simulink model "ROBOT4"  (R2019a)
settings: Solver=VariableStepAuto  StartTime=0.0  StopTime=inf  RelTol=1e-3
StartFcn:
  | 1
values from neighbouring files (symbols this model uses):
  s = sqrt((z4-a1)^2+r4^2)    [CONTROL.m]
undefined symbols (not defined in the file or in its folder): Base, Link1, Link2, Link3, Link4, ROBOT4, RootPart
libraries: mblibv1 x18, simulink x4
settings Model: Creator=MyPC  LastModifiedBy=csank
settings DataIOCC: ReturnWorkspaceOutputs=off
settings OptimizationCC: BlockReduction=off
settings DebuggingCC: ArithmeticOperatorsInVariantConditions=warning
settings SFSimCC: SimUseLocalCustomCode=off
settings RTWCC: RTWUseLocalCustomCode=off
settings CodeAppCC: StateflowObjectComments=on
settings SimscapeCC: SimscapeNormalizeSystem=off
settings SimMechanicsCC: VisOnUpdateDiagram=on  VisDuringSimulation=on

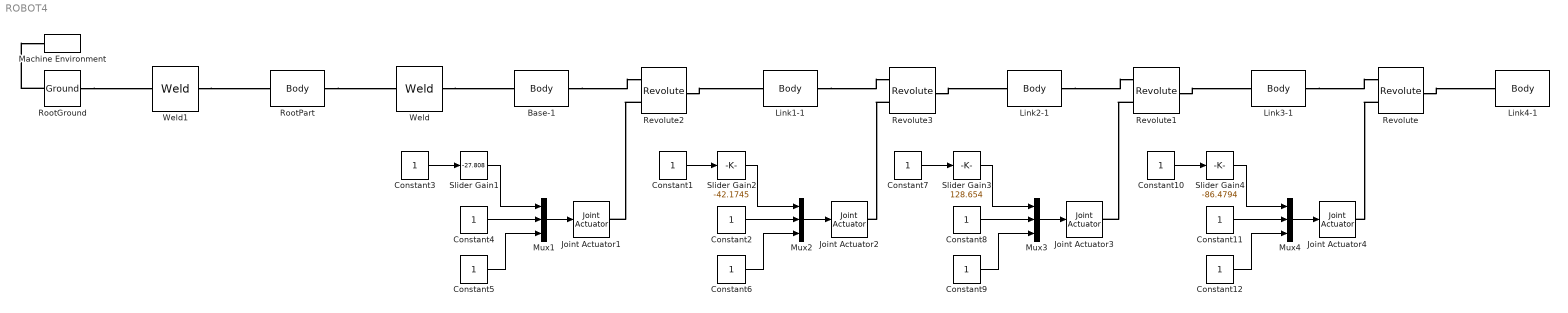
== system ROBOT4 ==
  Base-1 : mblibv1/Bodies/Body  LConnTagsString=CS2  RConnTagsString=CS3  UpdateFromCAD=on  PMImportedID=Base-1  DialogClass=MechanicalBodyBlock  Mass=20.055  MassUnits=kg  InertiaUnits=kg*m^2  Inertia=[0.425156,1.30045e-05,-3.32729e-05;1.30045e-05,0.499103,-0.0411844;-3.32729e-05,-0.0411844,0.340025]  Shape=Cylinder  ShapeDims=[1 1]  ShapeUnits=m  ShapeUse=false  Density=1  DensityUnits=kg/m^3  DensityUse=false  GraphicsMode=GFXFILE  GraphicsFileName=ROBOT4 - Base-1.STL  BodyColorSelMode=COLORPALETTE  BodyColor=[0.25098;0.25098;0.25098]  AttachedToCS=CS1  CG=Right$CG$[0.143839 0.24611 0.488748]$WORLD$WORLD$m$[1 0 0;0 1 0;0 0 1]$3x3 Transform$rad$WORLD$false$Base-1::CG(AUTOGEN)  WorkingFrames=Right$CS1$[0.143832 0.162841 0.457249]$WORLD$WORLD$m$[1 0 0;0 1 0;0 0 1]$3x3 Transform$rad$WORLD$false$Base-1::CS1(AUTOGEN)#Left$CS2$[0.143839 0.24611 0.488748]$WORLD$WORLD$m$[1 0 0;0 1 0;0 0 1]$3x3 Transform$rad$WORLD$true$Base-1:-:ROBOT4/RootPart::Base-1(AUTOGEN)#Right$CS3$[0.143832 0.312841 0.457249]$WORLD$WORLD$m$[1 0 0;0 1 0;0 0 1]$3x3 Transform$rad$WORLD$true$Base-1:-:Link1-1::Base-1(AUTOGEN)  CGPos=[0.143839 0.24611 0.488748]  CGRot=[1 0 0;0 1 0;0 0 1]  CS0Pos=[]  CS0Rot=[]  CS1Pos=[0.143832 0.162841 0.457249]  CS1Rot=[1 0 0;0 1 0;0 0 1]  CS2Pos=[0.143839 0.24611 0.488748]  CS2Rot=[1 0 0;0 1 0;0 0 1]  CS3Pos=[0.143832 0.312841 0.457249]  CS3Rot=[1 0 0;0 1 0;0 0 1]  CS4Pos=[]  CS4Rot=[]  CS5Pos=[]  CS5Rot=[]  CS6Pos=[]  CS6Rot=[]  CS7Pos=[]  CS7Rot=[]  CS8Pos=[]  CS8Rot=[]  CS9Pos=[]  CS9Rot=[]  CS10Pos=[]  CS10Rot=[]  CS11Pos=[]  CS11Rot=[]  CS12Pos=[]  CS12Rot=[]  CS13Pos=[]  CS13Rot=[]  CS14Pos=[]  CS14Rot=[]  CS15Pos=[]  CS15Rot=[]  CS16Pos=[]  CS16Rot=[]  CS17Pos=[]  CS17Rot=[]  CS18Pos=[]  CS18Rot=[]  CS19Pos=[]  CS19Rot=[]  CS20Pos=[]  CS20Rot=[]
      settings: SourceProductName=Simscape Multibody  SourceProductBaseCode=MS
  Constant{1..12} (12 alike) : Constant
  Joint Actuator{1..4} (4 alike) : mblibv1/Sensors &  Actuators/Joint Actuator  UpdateFromCAD=off  PhysicalDomain=Mechanical  PortType=blob  ActuationStyle=Motion  AngleUnits=deg  ArcVelocityUnits=deg/s  ArcAccelerationUnits=deg/s^2  CoordPositionUnits=m  VelocityUnits=m/s  AccelerationUnits=m/s^2  ForceUnits=N  TorqueUnits=N*m  ActiveIO=on  Width=3  DialogClass=MechanicalActuatorBlock  Primitive=R1  ReferenceFrame=Absolute (World)
      settings: SourceProductName=Simscape Multibody  SourceProductBaseCode=MS
  Link1-1 : mblibv1/Bodies/Body  LConnTagsString=CS2  RConnTagsString=CS3  UpdateFromCAD=on  PMImportedID=Link1-1  DialogClass=MechanicalBodyBlock  Mass=14.5082  MassUnits=kg  InertiaUnits=kg*m^2  Inertia=[0.281196,-1.21205e-09,1.25074e-09;-1.21205e-09,0.109377,0;1.25074e-09,0,0.307869]  Shape=Cylinder  ShapeDims=[1 1]  ShapeUnits=m  ShapeUse=false  Density=1  DensityUnits=kg/m^3  DensityUse=false  GraphicsMode=GFXFILE  GraphicsFileName=ROBOT4 - Link1-1.STL  BodyColorSelMode=COLORPALETTE  BodyColor=[0;0;1]  AttachedToCS=CS1  CG=Right$CG$[0.143832 0.525874 0.457249]$WORLD$WORLD$m$[0.791183 0 0.61158;0 1 0;-0.61158 0 0.791183]$3x3 Transform$rad$WORLD$false$Link1-1::CG(AUTOGEN)  WorkingFrames=Right$CS1$[0.143832 0.312841 0.457249]$WORLD$WORLD$m$[0.791183 0 0.61158;0 1 0;-0.61158 0 0.791183]$3x3 Transform$rad$WORLD$false$Link1-1::CS1(AUTOGEN)#Left$CS2$[0.143832 0.312841 0.457249]$WORLD$WORLD$m$[1 0 0;0 1 0;0 0 1]$3x3 Transform$rad$WORLD$true$Base-1:-:Link1-1::Link1-1(AUTOGEN)#Right$CS3$[0.0887895 0.648841 0.386043]$WORLD$WORLD$m$[1 0 0;0 1 0;0 0 1]$3x3 Transform$rad$WORLD$true$Link1-1:-:Link2-1::Link1-1(AUTOGEN)  CGPos=[0.143832 0.525874 0.457249]  CGRot=[0.791183 0 0.61158;0 1 0;-0.61158 0 0.791183]  CS0Pos=[]  CS0Rot=[]  CS1Pos=[0.143832 0.312841 0.457249]  CS1Rot=[0.791183 0 0.61158;0 1 0;-0.61158 0 0.791183]  CS2Pos=[0.143832 0.312841 0.457249]  CS2Rot=[1 0 0;0 1 0;0 0 1]  CS3Pos=[0.0887895 0.648841 0.386043]  CS3Rot=[1 0 0;0 1 0;0 0 1]  CS4Pos=[]  CS4Rot=[]  CS5Pos=[]  CS5Rot=[]  CS6Pos=[]  CS6Rot=[]  CS7Pos=[]  CS7Rot=[]  CS8Pos=[]  CS8Rot=[]  CS9Pos=[]  CS9Rot=[]  CS10Pos=[]  CS10Rot=[]  CS11Pos=[]  CS11Rot=[]  CS12Pos=[]  CS12Rot=[]  CS13Pos=[]  CS13Rot=[]  CS14Pos=[]  CS14Rot=[]  CS15Pos=[]  CS15Rot=[]  CS16Pos=[]  CS16Rot=[]  CS17Pos=[]  CS17Rot=[]  CS18Pos=[]  CS18Rot=[]  CS19Pos=[]  CS19Rot=[]  CS20Pos=[]  CS20Rot=[]
      settings: SourceProductName=Simscape Multibody  SourceProductBaseCode=MS
  Link2-1 : mblibv1/Bodies/Body  LConnTagsString=CS3  RConnTagsString=CS2  UpdateFromCAD=on  PMImportedID=Link2-1  DialogClass=MechanicalBodyBlock  Mass=15.1518  MassUnits=kg  InertiaUnits=kg*m^2  Inertia=[0.614194,-0.00012408,2.07767e-05;-0.00012408,0.151653,3.7792e-06;2.07767e-05,3.7792e-06,0.703306]  Shape=Cylinder  ShapeDims=[1 1]  ShapeUnits=m  ShapeUse=false  Density=1  DensityUnits=kg/m^3  DensityUse=false  GraphicsMode=GFXFILE  GraphicsFileName=ROBOT4 - Link2-1.STL  BodyColorSelMode=COLORPALETTE  BodyColor=[0;0;1]  AttachedToCS=CS1  CG=Right$CG$[0.293105 0.676583 0.341751]$WORLD$WORLD$m$[-0.61158 0.782776 0.11503;0 0.14539 -0.989374;-0.791183 -0.605082 -0.0889177]$3x3 Transform$rad$WORLD$false$Link2-1::CG(AUTOGEN)  WorkingFrames=Right$CS1$[0.143832 0.648841 0.457249]$WORLD$WORLD$m$[-0.61158 0.782776 0.11503;0 0.14539 -0.989374;-0.791183 -0.605082 -0.0889177]$3x3 Transform$rad$WORLD$false$Link2-1::CS1(AUTOGEN)#Right$CS2$[0.480177 0.721536 0.0835021]$WORLD$WORLD$m$[1 0 0;0 1 0;0 0 1]$3x3 Transform$rad$WORLD$true$Link2-1:-:Link3-1::Link2-1(AUTOGEN)#Left$CS3$[0.0887895 0.648841 0.386043]$WORLD$WORLD$m$[1 0 0;0 1 0;0 0 1]$3x3 Transform$rad$WORLD$true$Link1-1:-:Link2-1::Link2-1(AUTOGEN)  CGPos=[0.293105 0.676583 0.341751]  CGRot=[-0.61158 0.782776 0.11503;0 0.14539 -0.989374;-0.791183 -0.605082 -0.0889177]  CS0Pos=[]  CS0Rot=[]  CS1Pos=[0.143832 0.648841 0.457249]  CS1Rot=[-0.61158 0.782776 0.11503;0 0.14539 -0.989374;-0.791183 -0.605082 -0.0889177]  CS2Pos=[0.480177 0.721536 0.0835021]  CS2Rot=[1 0 0;0 1 0;0 0 1]  CS3Pos=[0.0887895 0.648841 0.386043]  CS3Rot=[1 0 0;0 1 0;0 0 1]  CS4Pos=[]  CS4Rot=[]  CS5Pos=[]  CS5Rot=[]  CS6Pos=[]  CS6Rot=[]  CS7Pos=[]  CS7Rot=[]  CS8Pos=[]  CS8Rot=[]  CS9Pos=[]  CS9Rot=[]  CS10Pos=[]  CS10Rot=[]  CS11Pos=[]  CS11Rot=[]  CS12Pos=[]  CS12Rot=[]  CS13Pos=[]  CS13Rot=[]  CS14Pos=[]  CS14Rot=[]  CS15Pos=[]  CS15Rot=[]  CS16Pos=[]  CS16Rot=[]  CS17Pos=[]  CS17Rot=[]  CS18Pos=[]  CS18Rot=[]  CS19Pos=[]  CS19Rot=[]  CS20Pos=[]  CS20Rot=[]
      settings: SourceProductName=Simscape Multibody  SourceProductBaseCode=MS
  Link3-1 : mblibv1/Bodies/Body  LConnTagsString=CS3  RConnTagsString=CS2  UpdateFromCAD=on  PMImportedID=Link3-1  DialogClass=MechanicalBodyBlock  Mass=11.44  MassUnits=kg  InertiaUnits=kg*m^2  Inertia=[0.316807,0,0;0,0.0703346,0.0335673;0,0.0335673,0.293359]  Shape=Cylinder  ShapeDims=[1 1]  ShapeUnits=m  ShapeUse=false  Density=1  DensityUnits=kg/m^3  DensityUse=false  GraphicsMode=GFXFILE  GraphicsFileName=ROBOT4 - Link3-1.STL  BodyColorSelMode=COLORPALETTE  BodyColor=[0;0;1]  AttachedToCS=CS1  CG=Right$CG$[0.65417 0.825127 0.0627608]$WORLD$WORLD$m$[-0.61158 0.783362 -0.110968;0 -0.140256 -0.990115;-0.791183 -0.605535 0.0857777]$3x3 Transform$rad$WORLD$false$Link3-1::CG(AUTOGEN)  WorkingFrames=Right$CS1$[0.53522 0.721536 0.154709]$WORLD$WORLD$m$[-0.61158 0.783362 -0.110968;0 -0.140256 -0.990115;-0.791183 -0.605535 0.0857777]$3x3 Transform$rad$WORLD$false$Link3-1::CS1(AUTOGEN)#Right$CS2$[0.891317 0.809701 -0.0573564]$WORLD$WORLD$m$[1 0 0;0 1 0;0 0 1]$3x3 Transform$rad$WORLD$true$Link3-1:-:Link4-1::Link3-1(AUTOGEN)#Left$CS3$[0.480177 0.721536 0.0835021]$WORLD$WORLD$m$[1 0 0;0 1 0;0 0 1]$3x3 Transform$rad$WORLD$true$Link2-1:-:Link3-1::Link3-1(AUTOGEN)  CGPos=[0.65417 0.825127 0.0627608]  CGRot=[-0.61158 0.783362 -0.110968;0 -0.140256 -0.990115;-0.791183 -0.605535 0.0857777]  CS0Pos=[]  CS0Rot=[]  CS1Pos=[0.53522 0.721536 0.154709]  CS1Rot=[-0.61158 0.783362 -0.110968;0 -0.140256 -0.990115;-0.791183 -0.605535 0.0857777]  CS2Pos=[0.891317 0.809701 -0.0573564]  CS2Rot=[1 0 0;0 1 0;0 0 1]  CS3Pos=[0.480177 0.721536 0.0835021]  CS3Rot=[1 0 0;0 1 0;0 0 1]  CS4Pos=[]  CS4Rot=[]  CS5Pos=[]  CS5Rot=[]  CS6Pos=[]  CS6Rot=[]  CS7Pos=[]  CS7Rot=[]  CS8Pos=[]  CS8Rot=[]  CS9Pos=[]  CS9Rot=[]  CS10Pos=[]  CS10Rot=[]  CS11Pos=[]  CS11Rot=[]  CS12Pos=[]  CS12Rot=[]  CS13Pos=[]  CS13Rot=[]  CS14Pos=[]  CS14Rot=[]  CS15Pos=[]  CS15Rot=[]  CS16Pos=[]  CS16Rot=[]  CS17Pos=[]  CS17Rot=[]  CS18Pos=[]  CS18Rot=[]  CS19Pos=[]  CS19Rot=[]  CS20Pos=[]  CS20Rot=[]
      settings: SourceProductName=Simscape Multibody  SourceProductBaseCode=MS
  Link4-1 : mblibv1/Bodies/Body  LConnTagsString=CS2  UpdateFromCAD=on  PMImportedID=Link4-1  DialogClass=MechanicalBodyBlock  Mass=1.35899  MassUnits=kg  InertiaUnits=kg*m^2  Inertia=[0.00780395,1.96668e-09,2.46591e-09;1.96668e-09,0.00251605,2.02055e-09;2.46591e-09,2.02055e-09,0.00833468]  Shape=Cylinder  ShapeDims=[1 1]  ShapeUnits=m  ShapeUse=false  Density=1  DensityUnits=kg/m^3  DensityUse=false  GraphicsMode=GFXFILE  GraphicsFileName=ROBOT4 - Link4-1.STL  BodyColorSelMode=COLORPALETTE  BodyColor=[1;1;1]  AttachedToCS=CS1  CG=Right$CG$[0.857915 0.812027 -0.0947335]$WORLD$WORLD$m$[-0.432065 -0.662789 -0.61158;-0.83772 0.5461 0;0.333984 0.512333 -0.791183]$3x3 Transform$rad$WORLD$false$Link4-1::CG(AUTOGEN)  WorkingFrames=Right$CS1$[0.940273 0.744169 -0.158395]$WORLD$WORLD$m$[-0.432065 -0.662789 -0.61158;-0.83772 0.5461 0;0.333984 0.512333 -0.791183]$3x3 Transform$rad$WORLD$false$Link4-1::CS1(AUTOGEN)#Left$CS2$[0.891317 0.809701 -0.0573564]$WORLD$WORLD$m$[1 0 0;0 1 0;0 0 1]$3x3 Transform$rad$WORLD$true$Link3-1:-:Link4-1::Link4-1(AUTOGEN)  CGPos=[0.857915 0.812027 -0.0947335]  CGRot=[-0.432065 -0.662789 -0.61158;-0.83772 0.5461 0;0.333984 0.512333 -0.791183]  CS0Pos=[]  CS0Rot=[]  CS1Pos=[0.940273 0.744169 -0.158395]  CS1Rot=[-0.432065 -0.662789 -0.61158;-0.83772 0.5461 0;0.333984 0.512333 -0.791183]  CS2Pos=[0.891317 0.809701 -0.0573564]  CS2Rot=[1 0 0;0 1 0;0 0 1]  CS3Pos=[]  CS3Rot=[]  CS4Pos=[]  CS4Rot=[]  CS5Pos=[]  CS5Rot=[]  CS6Pos=[]  CS6Rot=[]  CS7Pos=[]  CS7Rot=[]  CS8Pos=[]  CS8Rot=[]  CS9Pos=[]  CS9Rot=[]  CS10Pos=[]  CS10Rot=[]  CS11Pos=[]  CS11Rot=[]  CS12Pos=[]  CS12Rot=[]  CS13Pos=[]  CS13Rot=[]  CS14Pos=[]  CS14Rot=[]  CS15Pos=[]  CS15Rot=[]  CS16Pos=[]  CS16Rot=[]  CS17Pos=[]  CS17Rot=[]  CS18Pos=[]  CS18Rot=[]  CS19Pos=[]  CS19Rot=[]  CS20Pos=[]  CS20Rot=[]
      settings: SourceProductName=Simscape Multibody  SourceProductBaseCode=MS
  Machine Environment : mblibv1/Bodies/Machine Environment  PortType=env  PhysicalDomain=Mechanical  DialogTemplateClass=MECH.MachineEnvironment  SyncWhenCopied=off  Gravity=[0 -9.81 0]  GravityUnits=m/s^2  GravityAsSignal=off  Dimensionality=Auto-detect  AnalysisType=Forward dynamics  LinearAssemblyTolerance=1e-3  LinearAssemblyToleranceUnits=m  AngularAssemblyTolerance=1e-3  AngularAssemblyToleranceUnits=rad  ConstraintSolverType=Stabilizing  ConstraintRelTolerance=1e-4  ConstraintAbsTolerance=1e-4  UseRobustSingularityHandling=off  RedundancyAnalysisToleranceType=Automatically select tolerance  RedundancyAnalysisTolerance=1e-14  StatePerturbationType=Fixed  PerturbationSize=1e-5  VisualizeMachine=on  BodyVisualizationType=Use model default body geometries  BodyColorSelMode=Use model default  DefaultBodyColor=[1 0 0]
      settings: SourceProductName=Simscape Multibody  SourceProductBaseCode=MS
  Mux{1..4} (4 alike) : Mux  Inputs=3
  Revolute : mblibv1/Joints/Revolute  LConnTagsString=__newl0|SA1  RConnTagsString=__newr0  UpdateFromCAD=on  PMImportedID=Link3-1:-:Link4-1  NumSAPorts=1  CutJoint=off  MarkAsCut=off  Primitives=prismatic  PrimitiveProps=R1$World$[-0.61158,0,-0.791183]$revolute  DialogClass=JointBlock  R1Axis=[-0.61158,0,-0.791183]
      settings: SourceProductName=Simscape Multibody  SourceProductBaseCode=MS
  Revolute1 : mblibv1/Joints/Revolute  LConnTagsString=__newl0|SA1  RConnTagsString=__newr0  UpdateFromCAD=on  PMImportedID=Link2-1:-:Link3-1  NumSAPorts=1  CutJoint=off  MarkAsCut=off  Primitives=prismatic  PrimitiveProps=R1$World$[0.61158,0,0.791183]$revolute  DialogClass=JointBlock  R1Axis=[0.61158,0,0.791183]
      settings: SourceProductName=Simscape Multibody  SourceProductBaseCode=MS
  Revolute2 : mblibv1/Joints/Revolute  LConnTagsString=__newl0|SA1  RConnTagsString=__newr0  UpdateFromCAD=on  PMImportedID=Base-1:-:Link1-1  NumSAPorts=1  CutJoint=off  MarkAsCut=off  Primitives=prismatic  PrimitiveProps=R1$World$[0,1,0]$revolute  DialogClass=JointBlock  R1Axis=[0,1,0]
      settings: SourceProductName=Simscape Multibody  SourceProductBaseCode=MS
  Revolute3 : mblibv1/Joints/Revolute  LConnTagsString=__newl0|SA1  RConnTagsString=__newr0  UpdateFromCAD=on  PMImportedID=Link1-1:-:Link2-1  NumSAPorts=1  CutJoint=off  MarkAsCut=off  Primitives=prismatic  PrimitiveProps=R1$World$[-0.61158,0,-0.791183]$revolute  DialogClass=JointBlock  R1Axis=[-0.61158,0,-0.791183]
      settings: SourceProductName=Simscape Multibody  SourceProductBaseCode=MS
  RootGround : mblibv1/Bodies/Ground  UpdateFromCAD=on  PMImportedID=RootGround  LeftPortType=env  RightPortType=workingframe  PhysicalDomain=Mechanical  DialogClass=GroundBlock  CoordPosition=[0.288929,0.533635,0.35517]  CoordPositionUnits=m  StateVectorMgrId=0  MachineId=[1 0]  ShowEnvPort=on  ParameterChecksum=[2237965960, 2493805458, 3117988158, 3002818646]  TopologyChecksum=[2414812317, 896225707, 3049100628, 567793257]
      settings: SourceProductName=Simscape Multibody  SourceProductBaseCode=MS
  RootPart : mblibv1/Bodies/Body  LConnTagsString=CS3  RConnTagsString=CS2  UpdateFromCAD=on  PMImportedID=ROBOT4/RootPart  DialogClass=MechanicalBodyBlock  Mass=0  MassUnits=kg  InertiaUnits=kg*m^2  Inertia=[0,0,0;0,0,0;0,0,0]  Shape=Cylinder  ShapeDims=[1 1]  ShapeUnits=m  ShapeUse=false  Density=1  DensityUnits=kg/m^3  DensityUse=false  GraphicsMode=MACHINE_DEFAULT  BodyColorSelMode=MACHINE_DEFAULT  BodyColor=[1;0;0]  AttachedToCS=CS1  CG=Right$CG$[0.288929 0.533635 0.35517]$WORLD$WORLD$m$[1 0 0;0 1 0;0 0 1]$3x3 Transform$rad$WORLD$false$ROBOT4/RootPart::CG(AUTOGEN)  WorkingFrames=Right$CS1$[0 0 0]$WORLD$WORLD$m$[1 0 0;0 1 0;0 0 1]$3x3 Transform$rad$WORLD$false$ROBOT4/RootPart::CS1(AUTOGEN)#Right$CS2$[0.143839 0.24611 0.488748]$WORLD$WORLD$m$[1 0 0;0 1 0;0 0 1]$3x3 Transform$rad$WORLD$true$Base-1:-:ROBOT4/RootPart::ROBOT4/RootPart(AUTOGEN)#Left$CS3$[0.288929 0.533635 0.35517]$WORLD$WORLD$m$[1 0 0;0 1 0;0 0 1]$3x3 Transform$rad$WORLD$true$ROBOT4/RootPart:-:RootGround::ROBOT4/RootPart(AUTOGEN)  CGPos=[0.288929 0.533635 0.35517]  CGRot=[1 0 0;0 1 0;0 0 1]  CS0Pos=[]  CS0Rot=[]  CS1Pos=[0 0 0]  CS1Rot=[1 0 0;0 1 0;0 0 1]  CS2Pos=[0.143839 0.24611 0.488748]  CS2Rot=[1 0 0;0 1 0;0 0 1]  CS3Pos=[0.288929 0.533635 0.35517]  CS3Rot=[1 0 0;0 1 0;0 0 1]  CS4Pos=[]  CS4Rot=[]  CS5Pos=[]  CS5Rot=[]  CS6Pos=[]  CS6Rot=[]  CS7Pos=[]  CS7Rot=[]  CS8Pos=[]  CS8Rot=[]  CS9Pos=[]  CS9Rot=[]  CS10Pos=[]  CS10Rot=[]  CS11Pos=[]  CS11Rot=[]  CS12Pos=[]  CS12Rot=[]  CS13Pos=[]  CS13Rot=[]  CS14Pos=[]  CS14Rot=[]  CS15Pos=[]  CS15Rot=[]  CS16Pos=[]  CS16Rot=[]  CS17Pos=[]  CS17Rot=[]  CS18Pos=[]  CS18Rot=[]  CS19Pos=[]  CS19Rot=[]  CS20Pos=[]  CS20Rot=[]
      settings: SourceProductName=Simscape Multibody  SourceProductBaseCode=MS
  Slider Gain1 : simulink/Math Operations/Slider Gain  gain=-27.808  low=-180  high=180
  Slider Gain2 : simulink/Math Operations/Slider Gain  gain=-42.1745  low=-180  high=180
  Slider Gain3 : simulink/Math Operations/Slider Gain  gain=128.654  low=-180  high=180
  Slider Gain4 : simulink/Math Operations/Slider Gain  gain=-86.4794  low=-180  high=180
  Weld : mblibv1/Joints/Weld  LConnTagsString=__newl0  RConnTagsString=__newr0  UpdateFromCAD=on  PMImportedID=Base-1:-:ROBOT4/RootPart  NumSAPorts=0  CutJoint=off  MarkAsCut=off  Primitives=weld  PrimitiveProps=W$WORLD$[0.57735,0.57735,0.57735]$weld  DialogClass=JointBlock  WAxis=[0.57735,0.57735,0.57735]
      settings: SourceProductName=Simscape Multibody  SourceProductBaseCode=MS
  Weld1 : mblibv1/Joints/Weld  LConnTagsString=__newl0  RConnTagsString=__newr0  UpdateFromCAD=on  PMImportedID=ROBOT4/RootPart:-:RootGround  NumSAPorts=0  CutJoint=off  MarkAsCut=off  Primitives=weld  PrimitiveProps=W$WORLD$[0.57735,0.57735,0.57735]$weld  DialogClass=JointBlock  WAxis=[0.57735,0.57735,0.57735]
      settings: SourceProductName=Simscape Multibody  SourceProductBaseCode=MS
  wires:
  Slider Gain1/1 -> Mux1/1
  Mux1/1 -> Joint Actuator1/1
  Constant3/1 -> Slider Gain1/1
  Constant5/1 -> Mux1/3
  Constant4/1 -> Mux1/2
  Slider Gain2/1 -> Mux2/1
  Mux2/1 -> Joint Actuator2/1
  Constant1/1 -> Slider Gain2/1
  Constant6/1 -> Mux2/3
  Constant2/1 -> Mux2/2
  Slider Gain3/1 -> Mux3/1
  Mux3/1 -> Joint Actuator3/1
  Constant7/1 -> Slider Gain3/1
  Constant9/1 -> Mux3/3
  Constant8/1 -> Mux3/2
  Slider Gain4/1 -> Mux4/1
  Mux4/1 -> Joint Actuator4/1
  Constant10/1 -> Slider Gain4/1
  Constant12/1 -> Mux4/3
  Constant11/1 -> Mux4/2
  connections:
  RootPart/RConn1 -- Weld/LConn1
  Weld/RConn1 -- Base-1/LConn1
  Link3-1/RConn1 -- Revolute/LConn1
  Revolute/RConn1 -- Link4-1/LConn1
  Link2-1/RConn1 -- Revolute1/LConn1
  Revolute1/RConn1 -- Link3-1/LConn1
  Base-1/RConn1 -- Revolute2/LConn1
  Revolute2/RConn1 -- Link1-1/LConn1
  Link1-1/RConn1 -- Revolute3/LConn1
  Revolute3/RConn1 -- Link2-1/LConn1
  RootGround/RConn1 -- Weld1/LConn1
  Weld1/RConn1 -- RootPart/LConn1
  RootGround/LConn1 -- Machine Environment/RConn1
  Revolute2/LConn2 -- Joint Actuator1/RConn1
  Revolute3/LConn2 -- Joint Actuator2/RConn1
  Revolute1/LConn2 -- Joint Actuator3/RConn1
  Revolute/LConn2 -- Joint Actuator4/RConn1
